simulink model "Sum5"  (R2020b)
settings: Solver=VariableStepAuto  StartTime=0.0  StopTime=10.0  RelTol=1e-3
PreLoadFcn:
  | clc;
  | close all;
  | clear all;
  | R=10;
  | C=0.00001;
settings Model: Creator=Aradhana desai  LastModifiedBy=Aradhana desai

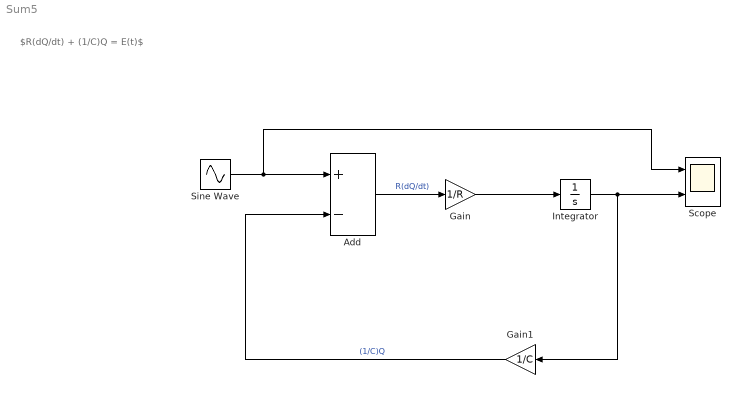
== system Sum5 ==
  note: $R(dQ/dt) + (1/C)Q = E(t)$
  Add : Sum  Inputs=+-
  Gain : Gain  Gain=1/R
  Gain1 : Gain  Gain=1/C
  Integrator : Integrator
  Scope : Scope  NumInputPorts=2
  Sine Wave : Sin  SampleTime=0
  wires:
  Sine Wave/1 -> Scope/1, Add/1
  Add/1 -> Gain/1  "R(dQ/dt)"
  Gain/1 -> Integrator/1
  Integrator/1 -> Gain1/1, Scope/2
  Gain1/1 -> Add/2  "(1/C)Q"
